simulink model "Tricopter_Controlled"  (R2015a)
settings: Solver=ode3  SolverMode=SingleTasking  StartTime=0.0  StopTime=inf  FixedStep=T_sim  RelTol=1e-3
values from neighbouring files (symbols this model uses):
  A_l_max_x = sqrt( (A_z_max)^2  -  g^2  )    [Run3Copter.m]
  A_l_max_y = g*tand(15)    [Run3Copter.m]
  A_z_max = Max_Thrust*3/m    [Run3Copter.m]
  Alt_0 = input(' Give the initial altitude (m): ')    [Run3Copter.m]
  B_hover_4dof = [-0.192641491537 -0.295051706147 -72.3190840892 -0.00308714144823 24.9504828653 -1.18743631629 9.87469464114e-05 6.48783896558 -0.0529805907426 -0.000387203135788 0.131620058452 2.24065603044 ... (54 elements, 6x9)]    [Effectiv_matrices.mat]
  CG_0 = [0,0,0.02]'    [SetupComplete.m]
  epsilon = 0.01    [Run3Copter.m]
  eta_23 = deg2rad(-1.3)    [Run3Copter.m]
  g = 9.81    [SetupComplete.m]
  h = 0.08    [SetupComplete.m]
  h_M = 0.064    [SetupComplete.m]
  Hover_eta_23 = deg2rad(-1.3)    [Run3Copter.m]
  Hover_throtle_1 = 0.745    [Run3Copter.m]
  Hover_throtle_23 = Hover_throtle_1/cos(Hover_eta_23)    [Run3Copter.m]
  I_BAC_0 = [ Ix,0,Ixz;0,Iy,0;Ixz,0,Iz]    [SetupComplete.m]
  Initial_Omegas = Omega_hover    [Run3Copter.m]
  Initial_Torques = Torque_hover    [Run3Copter.m]
  Ix = 0.103    [SetupComplete.m]
  Iy = 0.147    [SetupComplete.m]
  Iz = 0.237    [SetupComplete.m]
  l = 0.345    [SetupComplete.m]
  l_arm = 0.264    [SetupComplete.m]
  latitude = 52.071118    [Run3Copter.m]
  longitude = -0.627404    [Run3Copter.m]
  m = 3.51    [SetupComplete.m]
  m_0 = 2.61    [SetupComplete.m]
  m_M = 0.300    (= 0.3)    [SetupComplete.m]
  Rotation_sign = [ 1,-1,-1]    [SetupComplete.m]
  T_ctrl = 0.02    [Run3Copter.m]
  T_sim = 0.01    [Run3Copter.m]
  throtle_1 = 0*0.745    (= 0)    [Run3Copter.m]
  throtle_23 = throtle_1/cos(eta_23)    [Run3Copter.m]
  v_i0 = sqrt( 1/3*m*g/(2*rho*pi*R^2)  )    [SetupComplete.m]
undefined symbols (not defined in the file or in its folder): DOWN_0, EAST_0, Newton, NORTH_0, P_0, Q_0, R_0, Raphson, U_0, V_0, W_0
libraries: XXCopter_Control x64, simulink_extras x17, simulink x11, XXCopter x8
(part 3 of 6)

== system Tricopter_Controlled/TriCopter FCS/TriCopter FCS/Simulink_to_Px4 interface ==
  note: Terminal Debug Output
  note: RGB LED (uint8)
  note: Standard LED (Bool)
  note: PWM Output (uS)
  note: Enable Output (Bool)
  motors_signals : Inport
  servos_signals : Inport  Port=2
  pwm_arm : Inport  Port=3
  extern_signal_flihgt_mode : Inport  Port=4
  flight_mode : Inport  Port=5
  Bus Selector : BusSelector  OutputSignals=blue_LED,Red_LED,RGBLED.red,RGBLED.green,RGBLED.blue
  Data Type Conversion : DataTypeConversion  OutDataTypeStr=boolean
  Data Type Conversion1 : DataTypeConversion  OutDataTypeStr=boolean
  Data Type Conversion2 : DataTypeConversion  OutDataTypeStr=uint8
  Data Type Conversion3 : DataTypeConversion  OutDataTypeStr=uint8
  Data Type Conversion4 : DataTypeConversion  OutDataTypeStr=uint8
  Selector10 : Selector  InputPortWidth=6  Indices=4
  Selector11 : Selector  InputPortWidth=6  Indices=6
  Selector2 : Selector  InputPortWidth=3
  Selector3 : Selector  InputPortWidth=3  Indices=2
  Selector4 : Selector  InputPortWidth=3  Indices=3
  Selector5 : Selector  InputPortWidth=6  Indices=[1]
  Selector6 : Selector  InputPortWidth=6  Indices=[3]
  Selector8 : Selector  InputPortWidth=6  Indices=5
  Selector9 : Selector  InputPortWidth=6  Indices=[2]
  pwm1 : Outport  PortDimensions=1  SampleTime=T_ctrl
  pwm2 : Outport  Port=2  PortDimensions=1  SampleTime=T_ctrl
  pwm3 : Outport  Port=3  PortDimensions=1  SampleTime=T_ctrl
  pwm4 : Outport  Port=4  PortDimensions=1  SampleTime=T_ctrl
  pwm5 : Outport  Port=5  PortDimensions=1  SampleTime=T_ctrl
  pwm6 : Outport  Port=6  PortDimensions=1  SampleTime=T_ctrl
  pwm7 : Outport  Port=7  PortDimensions=1  SampleTime=T_ctrl
  pwm8 : Outport  Port=8  PortDimensions=1  SampleTime=T_ctrl
  pwm_arm1 : Outport  Port=9  PortDimensions=1  SampleTime=T_ctrl
  led_blue : Outport  Port=10  OutDataTypeStr=boolean  PortDimensions=1  SampleTime=T_ctrl
  led_red : Outport  Port=11  OutDataTypeStr=boolean  PortDimensions=1  SampleTime=T_ctrl
  rgb_red : Outport  Port=12  OutDataTypeStr=uint8  PortDimensions=1  SampleTime=T_ctrl
  rgb_green : Outport  Port=13  OutDataTypeStr=uint8  PortDimensions=1  SampleTime=T_ctrl
  rgb_blue : Outport  Port=14  OutDataTypeStr=uint8  PortDimensions=1  SampleTime=T_ctrl
  debug1 : Outport  Port=15  PortDimensions=1  SampleTime=T_ctrl
  debug2 : Outport  Port=16  PortDimensions=1  SampleTime=T_ctrl
  debug3 : Outport  Port=17  PortDimensions=1  SampleTime=T_ctrl
  debug4 : Outport  Port=18  PortDimensions=1  SampleTime=T_ctrl
  debug5 : Outport  Port=19  PortDimensions=1  SampleTime=T_ctrl
  debug6 : Outport  Port=20  PortDimensions=1  SampleTime=T_ctrl
  debug7 : Outport  Port=21  PortDimensions=1  SampleTime=T_ctrl
  debug8 : Outport  Port=22  PortDimensions=1  SampleTime=T_ctrl
  wires:
  motors_signals/1 -> Selector3/1, Selector4/1, Selector2/1
  servos_signals/1 -> Selector9/1, Selector5/1, Selector6/1, Selector10/1, Selector8/1, Selector11/1
  extern_signal_flihgt_mode/1 -> Bus Selector/1
  Bus Selector/2 -> Data Type Conversion1/1  "<Red_LED>"
  Selector2/1 -> pwm1/1
  Selector5/1 -> pwm2/1
  Selector9/1 -> pwm3/1
  Selector3/1 -> pwm4/1
  Selector6/1 -> pwm5/1
  Selector10/1 -> pwm6/1
  Selector4/1 -> pwm7/1
  Selector8/1 -> pwm8/1
  pwm_arm/1 -> pwm_arm1/1
  Bus Selector/3 -> Data Type Conversion2/1  "<red>"
  Bus Selector/4 -> Data Type Conversion3/1  "<green>"
  Bus Selector/5 -> Data Type Conversion4/1  "<blue>"
  flight_mode/1 -> debug8/1, debug7/1, debug6/1, debug5/1, debug4/1, debug3/1, debug1/1
  Data Type Conversion/1 -> led_blue/1
  Data Type Conversion1/1 -> led_red/1
  Data Type Conversion2/1 -> rgb_red/1
  Data Type Conversion3/1 -> rgb_green/1
  Data Type Conversion4/1 -> rgb_blue/1
  Selector11/1 -> debug2/1
  Bus Selector/1 -> Data Type Conversion/1  "<blue_LED>"

== system Tricopter_Controlled/TriCopter FCS/TriCopter FCS/Status signals ==
  flight_mode : Inport
  Not_allowed_change : Inport  Port=2
  Ground{,1..3} (4 alike) : Ground
  Beep : Outport
  Red_LED : Outport  Port=2
  blue_LED : Outport  Port=3
  blue_RGBLED : Outport  Port=4
  Red_RGBLED : Outport  Port=5
  green_RGBLED : Outport  Port=6
  wires:
  Ground/1 -> blue_RGBLED/1, Red_RGBLED/1, green_RGBLED/1
  Ground1/1 -> Beep/1
  Ground2/1 -> Red_LED/1
  Ground3/1 -> blue_LED/1

== system Tricopter_Controlled/TriCopter FCS/TriCopter FCS/flight_mode_effector ==
  flight_mode : Inport
  All_meas : Inport  Port=2
  Bus Creator : BusCreator  Inputs=6
  Bus Creator1 : BusCreator  Inputs=6
  Bus Selector1 : BusSelector  OutputSignals=Meas.Pos_meas_m,Params.V_yaw,Meas.Eulr_meas_rad,Meas.omega_b_meas_radps
  alt_act : Memory  X0=false  InheritSampleTime=on
  att_act : Memory  X0=false  InheritSampleTime=on
  flight_mode_effector : MATLAB Function  TreatAsAtomicUnit=on
  man_act : Memory  X0=false  InheritSampleTime=on
  pos_xy_act : Memory  X0=false  InheritSampleTime=on
  vel_yaw_xy_act : Memory  X0=false  InheritSampleTime=on
  vel_yaw_z_act : Memory  X0=false  InheritSampleTime=on
  Act_bus : Outport
  Controller_inits : Outport  Port=2  PortDimensions=12
  CA_reconf : Outport  Port=3
  Armed : Outport  Port=4
  wires:
  flight_mode/1 -> flight_mode_effector/1(flight_mode)
  flight_mode_effector/1(pos_xy_act) -> pos_xy_act/1
  flight_mode_effector/2(alt_act) -> alt_act/1
  flight_mode_effector/3(vel_yaw_xy_act) -> vel_yaw_xy_act/1
  flight_mode_effector/4(vel_yaw_z_act) -> vel_yaw_z_act/1
  flight_mode_effector/5(att_act) -> att_act/1
  flight_mode_effector/6(omega_b_act) -> man_act/1
  flight_mode_effector/9(vel_yaw_xy_init) -> Bus Creator1/3
  flight_mode_effector/12(b_rates_init) -> Bus Creator1/6
  flight_mode_effector/10(vel_yaw_z_init) -> Bus Creator1/4
  flight_mode_effector/11(att_init) -> Bus Creator1/5
  flight_mode_effector/7(pos_xy_init) -> Bus Creator1/1
  flight_mode_effector/8(alt_init) -> Bus Creator1/2
  Bus Selector1/2 -> flight_mode_effector/3(V_yaw)  "<V_yaw>"
  Bus Selector1/1 -> flight_mode_effector/2(X_e)  "<Pos_meas_m>"
  Bus Selector1/3 -> flight_mode_effector/4(Euler)  "<Eulr_meas_rad>"
  Bus Selector1/4 -> flight_mode_effector/5(omega_b)  "<omega_b_meas_radps>"
  pos_xy_act/1 -> Bus Creator/1  "pos_xy_act"
  alt_act/1 -> Bus Creator/2  "alt_act"
  vel_yaw_xy_act/1 -> Bus Creator/3  "vel_yaw_xy_act"
  vel_yaw_z_act/1 -> Bus Creator/4  "vel_yaw_z_act"
  att_act/1 -> Bus Creator/5  "att_act"
  man_act/1 -> Bus Creator/6  "omega_b_act"
  Bus Creator/1 -> Act_bus/1
  Bus Creator1/1 -> Controller_inits/1
  flight_mode_effector/13(CA_reconf) -> CA_reconf/1
  flight_mode_effector/14(Armed) -> Armed/1
  All_meas/1 -> Bus Selector1/1

== system Tricopter_Controlled/FlightGear visualization/Flat Earth to LLA/ne to lat//long/Latitude Between +//- 90  ==
  mu l : Inport
  Constant1 : Constant  Value=180
  Constant3 : Constant  Value=90
  Constant4 : Constant  Value=180
  Constant5 : Constant  Value=360
  Data Type Conversion : DataTypeConversion
  Demux : Demux  Outputs=2
  Gain : Gain  Gain=180
  Gain1 : Gain  Gain=2
  Gain2 : Gain  Gain=2
  Gain3 : Gain  Gain=360
  Gain4 : Gain  Gain=180
  Logical Operator1 : Logic  AllPortsSameDT=off  OutDataTypeStr=boolean
  Math Function1 : Math  Operator=rem  SaturateOnIntegerOverflow=on
  Math Function2 : Math  Operator=rem  SaturateOnIntegerOverflow=on
  Mux : Mux  Inputs=2
  Product : Product  Inputs=*/  RndMeth=Zero
  Product1 : Product  RndMeth=Zero
  Product2 : Product  Inputs=*/  RndMeth=Zero
  Product3 : Product  RndMeth=Zero
  Rounding Function : Rounding  Operator=fix
  Rounding Function1 : Rounding  Operator=fix
  Rounding Function2 : Rounding  Operator=fix
  Sum1 : Sum  Inputs=|-+
  Sum2 : Sum  Inputs=+--
  Sum3 : Sum  Inputs=++|
  sqrt : Sqrt  AlgorithmType=Newton-Raphson  SaturateOnIntegerOverflow=on
  "mu l " : Outport
  wires:
  Sum3/1 -> Mux/2
  Demux/2 -> Sum3/2
  Demux/1 -> Math Function1/1
  mu l/1 -> Demux/1
  Mux/1 -> "mu l "/1
  Constant1/1 -> Product/2
  Product/1 -> Rounding Function/1, Gain1/1
  Rounding Function/1 -> Gain/1
  Gain/1 -> Sum2/2
  Sum2/1 -> Mux/1
  Constant3/1 -> Math Function2/2
  Math Function2/1 -> Product3/2
  Product3/1 -> Sum2/3
  Rounding Function2/1 -> Gain2/1
  Gain2/1 -> Product3/1, Logical Operator1/1, Logical Operator1/2
  Product1/1 -> sqrt/1
  sqrt/1 -> Rounding Function2/1
  Constant4/1 -> Product2/2
  Product2/1 -> Rounding Function1/1
  Rounding Function1/1 -> Gain3/1
  Gain3/1 -> Sum1/1
  Math Function1/1 -> Sum1/2, Product2/1
  Sum1/1 -> Math Function2/1, Product/1, Sum2/1
  Constant5/1 -> Math Function1/2
  Logical Operator1/1 -> Data Type Conversion/1
  Gain4/1 -> Sum3/1
  Data Type Conversion/1 -> Gain4/1
  Gain1/1 -> Product1/2, Product1/1

== system Tricopter_Controlled/FlightGear visualization/Flat Earth to LLA/ne to lat//long/LongLat_offset  ==
  XY : Inport
  mu : Inport  Port=2
  " " : Trigonometry
  "  " : Trigonometry  Operator=cos
  Demux : Demux  Outputs=2
  "Find Radian/Distance " : Subsystem  TreatAsAtomicUnit=on
  Mux : Mux  Inputs=2
  Sum : Sum  Inputs=|+-
  Sum1 : Sum  Inputs=|++
  deg2rad : Gain  Gain=pi/180  SaturateOnIntegerOverflow=on  OutDataTypeStr=Inherit: Same as input  ParamDataTypeStr=Inherit: Same as input
  rad lat : Product  RndMeth=Zero
  "rad long " : Product  RndMeth=Zero
  ref_pos : Constant  Value=0
  x*cos : Product  RndMeth=Zero
  x*sin : Product  RndMeth=Zero
  y*cos : Product  RndMeth=Zero
  y*sin : Product  RndMeth=Zero
  DeltaLL_rad : Outport
  wires:
  mu/1 -> "Find Radian/Distance "/1(mu)
  "Find Radian/Distance "/1(dNorth) -> rad lat/2
  "Find Radian/Distance "/2(dEast) -> "rad long "/1
  rad lat/1 -> Mux/1
  "rad long "/1 -> Mux/2
  Mux/1 -> DeltaLL_rad/1
  deg2rad/1 -> "  "/1, " "/1
  Demux/2 -> y*cos/1, y*sin/1
  Sum1/1 -> "rad long "/2
  y*cos/1 -> Sum1/2
  x*sin/1 -> Sum1/1
  Sum/1 -> rad lat/1
  y*sin/1 -> Sum/2
  " "/1 -> x*sin/2, y*sin/2
  x*cos/1 -> Sum/1
  "  "/1 -> y*cos/2, x*cos/2
  Demux/1 -> x*sin/1, x*cos/1
  XY/1 -> Demux/1
  ref_pos/1 -> deg2rad/1

== system Tricopter_Controlled/FlightGear visualization/Flat Earth to LLA/ne to lat//long/Longitude Between +//-180  ==
  mu l : Inport
  Constant : Constant  Value=180
  Constant2 : Constant  Value=360
  Demux1 : Demux  Outputs=2
  Gain : Gain  Gain=360
  Math Function2 : Math  Operator=rem  SaturateOnIntegerOverflow=on
  Mux1 : Mux  Inputs=2
  Product : Product  Inputs=*/  RndMeth=Zero
  Rounding Function : Rounding  Operator=fix
  Sum2 : Sum  Inputs=|-+
  "mu l " : Outport
  wires:
  Mux1/1 -> "mu l "/1
  Demux1/1 -> Mux1/1
  mu l/1 -> Demux1/1
  Constant/1 -> Product/2
  Product/1 -> Rounding Function/1
  Rounding Function/1 -> Gain/1
  Gain/1 -> Sum2/1
  Sum2/1 -> Mux1/2
  Demux1/2 -> Math Function2/1
  Constant2/1 -> Math Function2/2
  Math Function2/1 -> Product/1, Sum2/2

== system Tricopter_Controlled/TriCopter FCS/Simulink to px4 input/Flat Earth to LLA/ne to lat//long ==
  Xe : Inport
  Demux : Demux  Outputs=2
  "Latitude Between +/- 90 " : Subsystem  TreatAsAtomicUnit=on
  "LongLat_offset " : Subsystem  TreatAsAtomicUnit=on
  "Longitude Between +/-180 " : Subsystem  TreatAsAtomicUnit=on
  Sel1 : Selector  InputPortWidth=3  Indices=[1,2]
  Sum2 : Sum  Inputs=++|
  initial_latg : Constant  Value=latitude
  initial_pos : Constant  Value=[latitude,longitude]
  rad2deg : Gain  Gain=180/pi  SaturateOnIntegerOverflow=on  OutDataTypeStr=Inherit: Same as input  ParamDataTypeStr=Inherit: Same as input
  lat_deg : Outport
  long_deg : Outport  Port=2
  wires:
  Xe/1 -> Sel1/1
  Sum2/1 -> "Latitude Between +/- 90 "/1(mu l)
  "LongLat_offset "/1(DeltaLL_rad) -> rad2deg/1
  Sel1/1 -> "LongLat_offset "/1(XY)
  rad2deg/1 -> Sum2/2
  initial_pos/1 -> Sum2/1
  initial_latg/1 -> "LongLat_offset "/2(mu)
  "Latitude Between +/- 90 "/1("mu l ") -> "Longitude Between +/-180 "/1(mu l)
  "Longitude Between +/-180 "/1("mu l ") -> Demux/1
  Demux/1 -> lat_deg/1
  Demux/2 -> long_deg/1

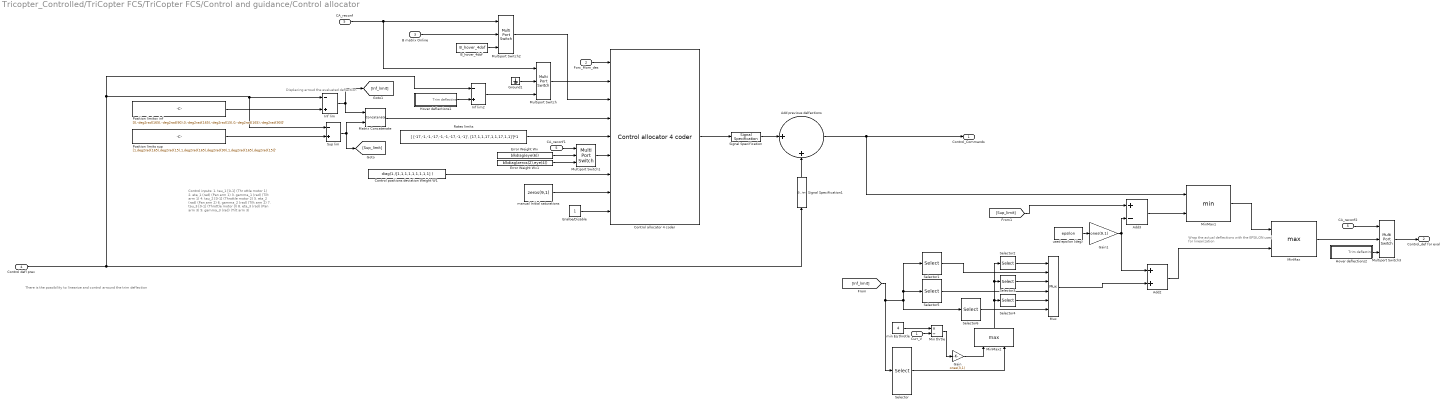
== system Tricopter_Controlled/TriCopter FCS/TriCopter FCS/Control and guidance/Control allocator ==
  note: There is the possibility to linearize and control arround the trim deflection
  note: Wrap the actual deflections with the EPSILON
      |  used for linearization
  note: Displacing arroud the evaluated deflection
  note: Control inputs:
      | 1. tau_1 [0-1] (Thr ottle motor 1)
      | 2. eta_1 (rad)  (Pan arm 1)
      | 3. gamma_1 (rad)  (Tilt arm 1)
      |
      | 4. tau_2 [0-1] (Throttle motor 2)
      | 5. eta_2 (rad)  (Pan arm 2)
      | 6. gamma_2 (rad)  (Tilt arm 2)
      |
      | 7. tau_3 [0-1] (Throttle motor 3)
      | 8. eta_3 (rad)  (Pan arm  3)
      | 9. gamma_3 (rad)  (Tilt arm 3)
  Curr_V : Inport
  Forc_Mom_des : Inport  Port=2
  B matrix Online : Inport  Port=3
  Control defl prev : Inport  Port=4
  CA_reconf : Inport  Port=5
  Add previous delfections : Sum  Inputs=|++
  Add2 : Sum
  Add3 : Sum  Inputs=+-
  B_hover_4dof : Constant  Value=B_hover_4dof
  CA_reconf1 : InportShadow  Port=5
  CA_reconf2 : InportShadow  Port=5
  Control allocator 4 coder : XXCopter_Control/Control allocator 4 coder  gamma=1  imax=50  T=T_ctrl
  Control positions deviation Weight W1 : Constant  Value=diag(1./[1,1,1,1,1,1,1,1,1] )
  Enalbe/Disable : Constant
  Error Weight Wv : Constant  Value=blkdiag(eye(6))
  Error Weight Wv1 : Constant  Value=blkdiag(zeros(2),eye(4))
  Gain : Gain  Gain=ones(3,1)
  Gain1 : Gain  Gain=ones(9,1)
  Ground1 : Ground
  Hover deflections1 : Subsystem  TreatAsAtomicUnit=on
  Hover deflections2 : Subsystem  TreatAsAtomicUnit=on
  Inf lim : Sum  Inputs=-+
  Inf lim2 : Sum  Inputs=-+
  Matrix Concatenate : Concatenate  Mode=Multidimensional array  ConcatenateDimension=2
  Min thrtle : Product  Inputs=*/
  MinMax : MinMax  Function=max  Inputs=2
  MinMax1 : MinMax  Inputs=2
  MinMax2 : MinMax  Function=max  Inputs=2
  Multiport Switch{,1..3} (4 alike) : MultiPortSwitch  Inputs=2
  Mux : Mux  Inputs=[1,2,1,2,1,2]
  Position limits sup : Constant  Value=[1,deg2rad(165),deg2rad(15),1,deg2rad(165),deg2rad(90),1,deg2rad(165),deg2rad(15)]'
  Position limitsv inf : Constant  Value=[0,-deg2rad(165),-deg2rad(90),0,-deg2rad(165),-deg2rad(15),0,-deg2rad(165),-deg2rad(90)]'
  Rates limits : Constant  Value=[ [-17,-1,-1,-17,-1,-1,-17,-1,-1]', [17,1,1,17,1,1,17,1,1]']*1
  Selector : Selector  InputPortWidth=9  Indices=[1,4,7]
  Selector1 : Selector  InputPortWidth=9  Indices=[2,3]
  Selector2 : Selector  InputPortWidth=3
  Selector3 : Selector  InputPortWidth=3
  Selector4 : Selector  InputPortWidth=3
  Selector5 : Selector  InputPortWidth=9  Indices=[2,3]
  Selector6 : Selector  InputPortWidth=9  Indices=[2,3]
  Signal Specification : SignalSpecification  Dimensions=[9,1]
  Signal Specification1 : SignalSpecification  Dimensions=[9,1]
  Sup lim : Sum  Inputs=-+
  manual Initial saturations : Constant  Value=zeros(9,1)
  min Eq throtle : Constant  Value=4
  used epsilon (deg) : Constant  Value=epsilon
  Control_Commands : Outport
  Control_def for eval : Outport  Port=2
  wires:
  MinMax1/1 -> MinMax/1
  Add3/1 -> MinMax1/2
  used epsilon (deg)/1 -> Gain1/1
  Gain1/1 -> Add2/1, Add3/2
  Add2/1 -> MinMax/2
  Control positions deviation Weight W1/1 -> Control allocator 4 coder/7
  Control allocator 4 coder/1 -> Signal Specification/1
  Enalbe/Disable/1 -> Control allocator 4 coder/9
  manual Initial saturations/1 -> Control allocator 4 coder/8
  Sup lim/1 -> [Sup_limit], Matrix Concatenate/2
  Inf lim/1 -> [Inf_limit], Matrix Concatenate/1
  Position limitsv inf/1 -> Inf lim/2
  Position limits sup/1 -> Sup lim/2
  Rates limits/1 -> Control allocator 4 coder/5
  Add previous delfections/1 -> Control_Commands/1, MinMax1/1
  Multiport Switch2/1 -> Control allocator 4 coder/3
  Signal Specification/1 -> Add previous delfections/1
  Signal Specification1/1 -> Add previous delfections/2
  Forc_Mom_des/1 -> Control allocator 4 coder/1
  Matrix Concatenate/1 -> Control allocator 4 coder/4
  Multiport Switch/1 -> Control allocator 4 coder/2
  Control defl prev/1 -> Signal Specification1/1, Inf lim/1, Sup lim/1, Inf lim2/1
  CA_reconf/1 -> Multiport Switch2/1, Multiport Switch/1
  B matrix Online/1 -> Multiport Switch2/2
  Ground1/1 -> Multiport Switch/2
  Inf lim2/1 -> Multiport Switch/3
  Hover deflections1/1(Trim deflectins) -> Inf lim2/2
  Multiport Switch3/1 -> Control_def for eval/1
  CA_reconf2/1 -> Multiport Switch3/1
  Hover deflections2/1(Trim deflectins) -> Multiport Switch3/3
  MinMax/1 -> Multiport Switch3/2
  B_hover_4dof/1 -> Multiport Switch2/3
  Multiport Switch1/1 -> Control allocator 4 coder/6
  CA_reconf1/1 -> Multiport Switch1/1
  Error Weight Wv/1 -> Multiport Switch1/2
  Error Weight Wv1/1 -> Multiport Switch1/3
  [Inf_limit] -> Selector5/1, Selector1/1, Selector6/1, Selector/1
  Selector/1 -> MinMax2/2
  min Eq throtle/1 -> Min thrtle/1
  Curr_V/1 -> Min thrtle/2
  Min thrtle/1 -> Gain/1
  Gain/1 -> MinMax2/1
  Selector2/1 -> Mux/1
  MinMax2/1 -> Selector4/1, Selector3/1, Selector2/1
  Selector3/1 -> Mux/3
  Selector4/1 -> Mux/5
  Selector1/1 -> Mux/2
  Selector5/1 -> Mux/4
  Selector6/1 -> Mux/6
  Mux/1 -> Add2/2
  [Sup_limit] -> Add3/1

== system Tricopter_Controlled/TriCopter FCS/TriCopter FCS/Control and guidance/Inner PI Controller Quaternions ==
  Accels ref (m/s^2) : Inport
  Phi_ref (rad) : Inport  Port=2
  Theta_ref (rad) : Inport  Port=3
  Yaw_ref (rad) : Inport  Port=4
  omega_b_ref_radps : Inport  Port=5
  All meas : Inport  Port=6
  activation_bus : Inport  Port=7
  init_cond : Inport  Port=8
  Add : Sum
  Add1 : Sum  Inputs=+-
  Add2 : Sum  Inputs=+-
  All meas1 : InportShadow  Port=6
  Attitude Controller : Subsystem
  Body Rates Controller : Subsystem
  Bus Selector : BusSelector  OutputSignals=Meas.Eulr_meas_rad
  Bus Selector1 : BusSelector  OutputSignals=Meas.q_meas
  Bus Selector2 : BusSelector  OutputSignals=att_act,omega_b_act
  Demux : Demux  Outputs=3
  Get Quaternion from des euler : MATLAB Function  TreatAsAtomicUnit=on
  Limits in Ang accel : Subsystem  TreatAsAtomicUnit=on
  Logical Operator2 : Logic  Operator=NOT  IconShape=distinctive  AllPortsSameDT=off  OutDataTypeStr=boolean
  Logical Operator3 : Logic  IconShape=distinctive  AllPortsSameDT=off  OutDataTypeStr=boolean
  MATLAB Function : MATLAB Function  TreatAsAtomicUnit=on
  Memory : Memory
  Mux : Mux  Inputs=2
  Quaternion_dot : MATLAB Function  TreatAsAtomicUnit=on  VariantControl=Variant
  Saturation1 : Saturate  UpperLimit=deg2rad(50)*[1,10,0.5]'  LowerLimit=-deg2rad(50)*[1,10,0.5]'
  Switch1 : Switch  Criteria=u2 ~= 0
  T : Gain  Gain=T_ctrl
  Accs_Ang_acc des : Outport
  wires:
  Accels ref (m/s^2)/1 -> Mux/1
  Mux/1 -> Accs_Ang_acc des/1
  All meas/1 -> Bus Selector/1, Attitude Controller/5(All_meas)
  Bus Selector/1 -> Limits in Ang accel/2(Euler meas), MATLAB Function/2(Euler)  "<Eulr_meas_rad>"
  Demux/1 -> Body Rates Controller/1(p_ref)
  Demux/2 -> Body Rates Controller/2(q_ref)
  Demux/3 -> Body Rates Controller/3(r_ref)
  Phi_ref (rad)/1 -> Attitude Controller/2(Phi_ref (rad)), Get Quaternion from des euler/1(phi)
  Theta_ref (rad)/1 -> Get Quaternion from des euler/2(theta)
  Yaw_ref (rad)/1 -> Attitude Controller/4(Yaw_ref (rad)), Get Quaternion from des euler/3(psi)
  Bus Selector1/1 -> Quaternion_dot/2(q)  "<q_meas>"
  Get Quaternion from des euler/1(q) -> Attitude Controller/3(q_ref)
  Attitude Controller/1(quat_dot des (rad/s)) -> Quaternion_dot/1(q_dot)
  Limits in Ang accel/1(ang Ace des) -> Add2/1, Mux/2
  Switch1/1 -> Add1/2, Saturation1/1
  Body Rates Controller/1(Angular acc des (rad/s^2)) -> Add2/2, Limits in Ang accel/1(Ang Ace des)
  Add/1 -> MATLAB Function/1(omega_b)
  Add2/1 -> T/1
  Add1/1 -> Add/2
  T/1 -> Add/1
  MATLAB Function/1(Euler_dot) -> Memory/1
  init_cond/1 -> Body Rates Controller/5(init_cond), Attitude Controller/7(init_cond)
  activation_bus/1 -> Attitude Controller/6(activation_bus), Bus Selector2/1, Body Rates Controller/6(activation_bus)
  All meas1/1 -> Body Rates Controller/4(All_meas), Bus Selector1/1
  Bus Selector2/1 -> Logical Operator2/1  "<att_act>"
  Logical Operator2/1 -> Logical Operator3/1
  Bus Selector2/2 -> Logical Operator3/2  "<omega_b_act>"
  Saturation1/1 -> Demux/1, Add1/1
  Logical Operator3/1 -> Switch1/2
  Quaternion_dot/1(omega_b) -> Switch1/3
  omega_b_ref_radps/1 -> Switch1/1
  Memory/1 -> Attitude Controller/1(AWU)

== system Tricopter_Controlled/TriCopter FCS/TriCopter FCS/Control and guidance/NDI ==
  note: Rejection for the
      | angular accelerations
  note: Pseudo control inputs:
      | 1. Desired angular accelerations (rad/s^2)
      | 2. Desired accelerations (m/s^2) in body axes
  pseudo_control (m/s^2;rad/s^2) : Inport
  Control_defl for eval : Inport  Port=2
  All_meas : Inport  Port=3
  3Copter_4_NDI&CA : Subsystem  TreatAsAtomicUnit=on
  Bus Selector : BusSelector  OutputSignals=Meas.omega_b_meas_radps,Meas.q_meas,Meas.V_b_meas,Meas.Alt_meas_m,Meas.Volt
  Demux : Demux  Outputs=[3,3]
  Derivative1 : Derivative  CoefficientInTFapproximation=500
  Ground : Ground
  Ground1 : Ground
  Inversion : Sum  Inputs=|+-
  Mux : Mux  Inputs=[3,3]
  Mux2 : Mux  Inputs=[3,3]
  Rot eqs_ Get moments : XXCopter_Control/Rot eqs_ Get moments
  Transl Eqs_ Get forces : XXCopter_Control/Transl Eqs_ Get forces
  "angles " : Selector  IndexMode=Zero-based  InputPortWidth=9  Indices=[1,2,4,5,7,8]
  epsilon (rad or unitary) : Constant  Value=epsilon
  m : Constant  Value=m
  m1 : Constant  Value=m
  Virtual Control Commands : Outport
  B online : Outport  Port=2
  Control_defl eval (rad) : Outport  Port=3
  wires:
  3Copter_4_NDI&CA/3(CA_grad) -> B online/1
  Mux/1 -> Inversion/1
  Mux2/1 -> Inversion/2  "f_x(x)"
  All_meas/1 -> Bus Selector/1
  pseudo_control (m/s^2;rad/s^2)/1 -> Demux/1
  Demux/2 -> Rot eqs_ Get moments/2, Transl Eqs_ Get forces/4
  Demux/1 -> Transl Eqs_ Get forces/1
  Bus Selector/1 -> Transl Eqs_ Get forces/3, Rot eqs_ Get moments/1, 3Copter_4_NDI&CA/6(omega_b)  "<omega_b_meas_radps>"
  Bus Selector/3 -> Transl Eqs_ Get forces/2, 3Copter_4_NDI&CA/4(Vb)  "<V_b_meas>"
  3Copter_4_NDI&CA/4(I_BAC) -> Rot eqs_ Get moments/3
  3Copter_4_NDI&CA/5("CG ") -> Transl Eqs_ Get forces/6
  Control_defl for eval/1 -> 3Copter_4_NDI&CA/2(Control Inputs (rad)), Control_defl eval (rad)/1, "angles "/1
  Bus Selector/4 -> 3Copter_4_NDI&CA/3(h)  "<Alt_meas_m>"
  Bus Selector/2 -> 3Copter_4_NDI&CA/5(q)  "<q_meas>"
  m1/1 -> 3Copter_4_NDI&CA/11(" m")
  m/1 -> Transl Eqs_ Get forces/5
  epsilon (rad or unitary)/1 -> 3Copter_4_NDI&CA/1("epsilon (rad or unitary) ")
  Transl Eqs_ Get forces/1 -> Mux/1
  Rot eqs_ Get moments/1 -> Mux/2
  3Copter_4_NDI&CA/1(Forces) -> Mux2/1
  3Copter_4_NDI&CA/2(Moments) -> Mux2/2
  Inversion/1 -> Virtual Control Commands/1
  Ground/1 -> 3Copter_4_NDI&CA/7(Omegas_dot_actual)
  "angles "/1 -> Derivative1/1, 3Copter_4_NDI&CA/8(angles_actual)
  Derivative1/1 -> 3Copter_4_NDI&CA/9(angles_dot_actual)
  Ground1/1 -> 3Copter_4_NDI&CA/10(angles_dot_dot_actual)
  Bus Selector/5 -> 3Copter_4_NDI&CA/12(Curr_V)  "<Volt>"

== system Tricopter_Controlled/TriCopter FCS/TriCopter FCS/Control and guidance/Otter Overactuated P Controller ==
  Position ref (m) : Inport
  Vel_yaw_ref(m) : Inport  Port=2
  All meas : Inport  Port=3
  activation_bus : Inport  Port=4
  init_cond : Inport  Port=5
  AWU : Product  Multiplication=Matrix(*)
  Add : Sum
  Add1 : Sum  Inputs=+-
  Add2 : Sum  Inputs=+-
  Bus Selector1 : BusSelector  OutputSignals=Params.T_Fe_Fyaw,Params.V_yaw,Params.DCM
  Bus Selector2 : BusSelector  OutputSignals=pos_xy_act,vel_yaw_xy_act,alt_act,vel_yaw_z_act
  Demux1 : Demux  Outputs=3
  Demux2 : Demux  Outputs=3
  Demux3 : Demux  Outputs=[2,1]
  Logical Operator : Logic  IconShape=distinctive  AllPortsSameDT=off  OutDataTypeStr=boolean
  Logical Operator1 : Logic  Operator=NOT  IconShape=distinctive  AllPortsSameDT=off  OutDataTypeStr=boolean
  Logical Operator2 : Logic  Operator=NOT  IconShape=distinctive  AllPortsSameDT=off  OutDataTypeStr=boolean
  Logical Operator3 : Logic  IconShape=distinctive  AllPortsSameDT=off  OutDataTypeStr=boolean
  Matrix Multiply1 : Product  Multiplication=Matrix(*)
  Matrix Multiply2 : Product  Multiplication=Matrix(*)
  Matrix Multiply3 : Product  Multiplication=Matrix(*)
  Memory : Memory
  Mux : Mux  Inputs=[2,1]
  Permute Dimensions : PermuteDimensions
  Permute Dimensions1 : PermuteDimensions
  Permute Dimensions2 : PermuteDimensions
  Position Controller : Subsystem
  Saturation : Saturate  UpperLimit=[A_l_max_x,A_l_max_y,g]  LowerLimit=-[A_l_max_x,A_l_max_y,A_z_max-g]
  Saturation1 : Saturate  UpperLimit=[10,10,v_i0]'  LowerLimit=-[10,10,2*v_i0]'
  Selector : Selector  InputPortWidth=3  Indices=[1,2]
  Selector1 : Selector  InputPortWidth=3  Indices=3
  Switch : Switch  Criteria=u2 ~= 0
  Switch1 : Switch  Criteria=u2 ~= 0
  T : Gain  Gain=T_ctrl
  Velocity Controller : Subsystem
  activation_bus1 : InportShadow  Port=4
  init_cond1 : InportShadow  Port=5
  Accels des : Outport
  wires:
  Demux2/3 -> Velocity Controller/3(Vyaw_z_ref)
  Demux2/1 -> Velocity Controller/1(Vyaw_x_ref)
  Demux2/2 -> Velocity Controller/2(Vyaw_y_ref)
  All meas/1 -> Position Controller/6(All_meas), Bus Selector1/1
  Position ref (m)/1 -> Demux1/1
  Demux1/3 -> Position Controller/4(X_e_z_ref)
  Demux1/2 -> Position Controller/3(X_e_y_ref)
  Demux1/1 -> Position Controller/2(X_e_x_ref)
  Bus Selector1/3 -> Permute Dimensions/1  "<DCM>"
  Matrix Multiply1/1 -> Accels des/1
  Permute Dimensions/1 -> Matrix Multiply1/1
  Position Controller/1(Ve des (m/s)) -> Matrix Multiply2/2
  Saturation1/1 -> Add1/1, Demux2/1
  Saturation/1 -> Add2/1, Matrix Multiply3/2
  Bus Selector1/1 -> Permute Dimensions2/1, Matrix Multiply2/1, Permute Dimensions1/1  "<T_Fe_Fyaw>"
  Mux/1 -> Add1/2, Saturation1/1
  Matrix Multiply3/1 -> Matrix Multiply1/2  "in F_e"
  Permute Dimensions1/1 -> Matrix Multiply3/1
  Velocity Controller/1(Acc_yaw des (m/s)) -> Add2/2, Saturation/1
  Permute Dimensions2/1 -> AWU/1
  Add/1 -> AWU/2
  Add2/1 -> T/1
  Add1/1 -> Add/2
  AWU/1 -> Memory/1
  T/1 -> Add/1
  activation_bus/1 -> Bus Selector2/1, Position Controller/5(activation_bus)
  activation_bus1/1 -> Velocity Controller/5(activation_bus)
  init_cond/1 -> Position Controller/7(init_cond)
  Bus Selector1/2 -> Velocity Controller/4(V_yaw_meas)  "<V_yaw>"
  Matrix Multiply2/1 -> Demux3/1
  Switch/1 -> Mux/1
  Demux3/1 -> Switch/3
  Vel_yaw_ref(m)/1 -> Selector/1, Selector1/1
  Selector/1 -> Switch/1
  Switch1/1 -> Mux/2
  Demux3/2 -> Switch1/3
  Selector1/1 -> Switch1/1
  init_cond1/1 -> Velocity Controller/6(Init_cond)
  Bus Selector2/1 -> Logical Operator1/1  "<pos_xy_act>"
  Bus Selector2/3 -> Logical Operator2/1  "<alt_act>"
  Logical Operator1/1 -> Logical Operator/1
  Bus Selector2/2 -> Logical Operator/2  "<vel_yaw_xy_act>"
  Logical Operator2/1 -> Logical Operator3/1
  Bus Selector2/4 -> Logical Operator3/2  "<vel_yaw_z_act>"
  Logical Operator/1 -> Switch/2
  Logical Operator3/1 -> Switch1/2
  Memory/1 -> Position Controller/1(AWU)

== system Tricopter_Controlled/TriCopter FCS/TriCopter FCS/Control and guidance/keep -90//90 ==
  in (rad) : Inport
  Constant : Constant  Value=180
  Constant2 : Constant  Value=360
  Gain : Gain  Gain=360
  Math Function2 : Math  Operator=rem  SaturateOnIntegerOverflow=on
  Product : Product  Inputs=*/  RndMeth=Zero
  Rounding Function : Rounding  Operator=fix
  Sum2 : Sum  Inputs=|-+
  deg2rad1 : Gain  Gain=pi/180  SaturateOnIntegerOverflow=on  OutDataTypeStr=Inherit: Same as input  ParamDataTypeStr=Inherit: Same as input
  rad2deg : Gain  Gain=180/pi  SaturateOnIntegerOverflow=on  OutDataTypeStr=Inherit: Same as input  ParamDataTypeStr=Inherit: Same as input
  out (rad) : Outport
  wires:
  deg2rad1/1 -> out (rad)/1
  Sum2/1 -> deg2rad1/1
  Math Function2/1 -> Sum2/2, Product/1
  Constant2/1 -> Math Function2/2
  rad2deg/1 -> Math Function2/1
  Gain/1 -> Sum2/1
  Rounding Function/1 -> Gain/1
  Product/1 -> Rounding Function/1
  Constant/1 -> Product/2
  in (rad)/1 -> rad2deg/1

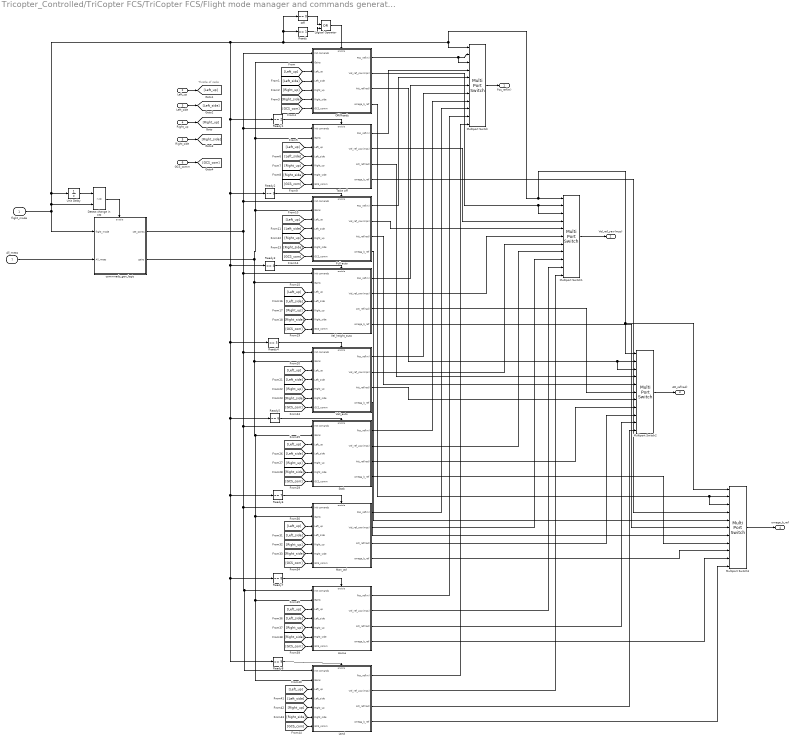
== system Tricopter_Controlled/TriCopter FCS/TriCopter FCS/Flight mode manager and commands generator/Commands generator ==
  note: Throtle of radio
  flight_mode : Inport
  Left_up : Inport  Port=2
  Left_side : Inport  Port=3
  Right_up : Inport  Port=4
  Right_side : Inport  Port=5
  GCS_comm : Inport  Port=6
  All_meas : Inport  Port=7
  Detect change in FM : RelationalOperator  Operator=~=  OutDataTypeStr=boolean
  Full auto : Subsystem  TreatAsAtomicUnit=on
  Home : Subsystem  TreatAsAtomicUnit=on
  "Land " : Subsystem  TreatAsAtomicUnit=on
  Logical Operator : Logic  Operator=OR  IconShape=distinctive  AllPortsSameDT=off  OutDataTypeStr=boolean
  Man_ctrl : Subsystem  TreatAsAtomicUnit=on
  Multiport Switch{,1..3} (4 alike) : MultiPortSwitch  DataPortOrder=Zero-based contiguous  Inputs=10
  Off : simulink/Logic and Bit Operations/Compare To Constant  relop===  const=0  OutDataTypeStr=boolean
  Off/Ready : Subsystem  TreatAsAtomicUnit=on
  Ready : simulink/Logic and Bit Operations/Compare To Constant  relop===  const=1  OutDataTypeStr=boolean
  Ready1 : simulink/Logic and Bit Operations/Compare To Constant  relop===  const=2  OutDataTypeStr=boolean
  Ready2 : simulink/Logic and Bit Operations/Compare To Constant  relop===  const=3  OutDataTypeStr=boolean
  Ready3 : simulink/Logic and Bit Operations/Compare To Constant  relop===  const=4  OutDataTypeStr=boolean
  Ready4 : simulink/Logic and Bit Operations/Compare To Constant  relop===  const=5  OutDataTypeStr=boolean
  Ready5 : simulink/Logic and Bit Operations/Compare To Constant  relop===  const=6  OutDataTypeStr=boolean
  Ready6 : simulink/Logic and Bit Operations/Compare To Constant  relop===  const=7  OutDataTypeStr=boolean
  Ready7 : simulink/Logic and Bit Operations/Compare To Constant  relop===  const=8  OutDataTypeStr=boolean
  Ready8 : simulink/Logic and Bit Operations/Compare To Constant  relop===  const=9  OutDataTypeStr=boolean
  Stab : Subsystem  TreatAsAtomicUnit=on
  Take off : Subsystem  TreatAsAtomicUnit=on
  Unit Delay : UnitDelay  SampleTime=-1
  Vel_height_auto : Subsystem  TreatAsAtomicUnit=on
  Vell_auto : Subsystem  TreatAsAtomicUnit=on
  commnads_gen_logic : Subsystem
  Pos_ref(m) : Outport
  Vel_ref_yaw(mps) : Outport  Port=2
  Att_ref(rad) : Outport  Port=3
  omega_b_ref : Outport  Port=4
  wires:
  flight_mode/1 -> Detect change in FM/2, Unit Delay/1, Ready8/1, Ready7/1, Ready6/1, Ready5/1, Ready4/1, Ready3/1, Ready2/1, Ready1/1, Ready/1, Off/1, Multiport Switch2/1, Multiport Switch3/1, Multiport Switch1/1, Multiport Switch/1, commnads_gen_logic/1(flight_mode)
  Multiport Switch/1 -> Pos_ref(m)/1
  Multiport Switch1/1 -> Vel_ref_yaw(mps)/1
  Multiport Switch2/1 -> Att_ref(rad)/1
  Multiport Switch3/1 -> omega_b_ref/1
  Right_up/1 -> [Right_up]
  Left_up/1 -> [Left_up]
  Right_side/1 -> [Right_side]
  Left_side/1 -> [Left_side]
  GCS_comm/1 -> [GCS_com]
  [Left_up] -> Off/Ready/3(Left_up)
  [Left_side] -> Off/Ready/4(Left_side)
  [Right_up] -> Off/Ready/5(Right_up)
  [Right_side] -> Off/Ready/6(Right_side)
  [GCS_com] -> Off/Ready/7(GCS_comm)
  [Left_up] -> Take off/3(Left_up)
  [Left_side] -> Take off/4(Left_side)
  [Right_up] -> Take off/5(Right_up)
  [Right_side] -> Take off/6(Right_side)
  [GCS_com] -> Take off/7(GCS_comm)
  [Left_up] -> Full auto/3(Left_up)
  [Left_side] -> Full auto/4(Left_side)
  [Right_up] -> Full auto/5(Right_up)
  [Right_side] -> Full auto/6(Right_side)
  [GCS_com] -> Full auto/7(GCS_comm)
  [Left_up] -> Vel_height_auto/3(Left_up)
  [Left_side] -> Vel_height_auto/4(Left_side)
  [Right_up] -> Vel_height_auto/5(Right_up)
  [Right_side] -> Vel_height_auto/6(Right_side)
  [GCS_com] -> Vel_height_auto/7(GCS_comm)
  [Left_up] -> Vell_auto/3(Left_up)
  [Left_side] -> Vell_auto/4(Left_side)
  [Right_up] -> Vell_auto/5(Right_up)
  [Right_side] -> Vell_auto/6(Right_side)
  [GCS_com] -> Vell_auto/7(GCS_comm)
  [Left_up] -> Stab/3(Left_up)
  [Left_side] -> Stab/4(Left_side)
  [Right_up] -> Stab/5(Right_up)
  [Right_side] -> Stab/6(Right_side)
  [GCS_com] -> Stab/7(GCS_comm)
  [Left_up] -> Man_ctrl/3(Left_up)
  [Left_side] -> Man_ctrl/4(Left_side)
  [Right_up] -> Man_ctrl/5(Right_up)
  [Right_side] -> Man_ctrl/6(Right_side)
  [GCS_com] -> Man_ctrl/7(GCS_comm)
  [Left_up] -> Home/3(Left_up)
  [Left_side] -> Home/4(Left_side)
  [Right_up] -> Home/5(Right_up)
  [Right_side] -> Home/6(Right_side)
  [GCS_com] -> Home/7(GCS_comm)
  [Left_up] -> "Land "/3(Left_up)
  [Left_side] -> "Land "/4(Left_side)
  [Right_up] -> "Land "/5(Right_up)
  [Right_side] -> "Land "/6(Right_side)
  [GCS_com] -> "Land "/7(GCS_comm)
  Off/1 -> Logical Operator/1
  Ready/1 -> Logical Operator/2
  Logical Operator/1 -> Off/Ready/Enable
  Ready1/1 -> Take off/Enable
  Ready2/1 -> Full auto/Enable
  Ready3/1 -> Vel_height_auto/Enable
  Ready4/1 -> Vell_auto/Enable
  Ready5/1 -> Stab/Enable
  Ready6/1 -> Man_ctrl/Enable
  Ready7/1 -> Home/Enable
  Ready8/1 -> "Land "/Enable
  Off/Ready/1(Pos_ref(m)) -> Multiport Switch/3, Multiport Switch/2
  Take off/1(Pos_ref(m)) -> Multiport Switch/4
  Full auto/1(Pos_ref(m)) -> Multiport Switch/5
  Vel_height_auto/1(Pos_ref(m)) -> Multiport Switch/6
  Vell_auto/1(Pos_ref(m)) -> Multiport Switch/7
  Stab/1(Pos_ref(m)) -> Multiport Switch/8
  Man_ctrl/1(Pos_ref(m)) -> Multiport Switch/9
  Home/1(Pos_ref(m)) -> Multiport Switch/10
  "Land "/1(Pos_ref(m)) -> Multiport Switch/11
  Off/Ready/2(Vel_ref_yaw(mps)) -> Multiport Switch1/3, Multiport Switch1/2
  Take off/2(Vel_ref_yaw(mps)) -> Multiport Switch1/4
  Full auto/2(Vel_ref_yaw(mps)) -> Multiport Switch1/5
  Vel_height_auto/2(Vel_ref_yaw(mps)) -> Multiport Switch1/6
  Vell_auto/2(Vel_ref_yaw(mps)) -> Multiport Switch1/7
  Stab/2(Vel_ref_yaw(mps)) -> Multiport Switch1/8
  Man_ctrl/2(Vel_ref_yaw(mps)) -> Multiport Switch1/9
  Home/2(Vel_ref_yaw(mps)) -> Multiport Switch1/10
  "Land "/2(Vel_ref_yaw(mps)) -> Multiport Switch1/11
  Off/Ready/3(Att_ref(rad)) -> Multiport Switch2/3, Multiport Switch2/2
  Take off/3(Att_ref(rad)) -> Multiport Switch2/4
  Full auto/3(Att_ref(rad)) -> Multiport Switch2/5
  Vel_height_auto/3(Att_ref(rad)) -> Multiport Switch2/6
  Vell_auto/3(Att_ref(rad)) -> Multiport Switch2/7
  Stab/3(Att_ref(rad)) -> Multiport Switch2/8
  Man_ctrl/3(Att_ref(rad)) -> Multiport Switch2/9
  Home/3(Att_ref(rad)) -> Multiport Switch2/10
  "Land "/3(Att_ref(rad)) -> Multiport Switch2/11
  Off/Ready/4(omega_b_ref) -> Multiport Switch3/3, Multiport Switch3/2
  Take off/4(omega_b_ref) -> Multiport Switch3/4
  Full auto/4(omega_b_ref) -> Multiport Switch3/5
  Vel_height_auto/4(omega_b_ref) -> Multiport Switch3/6
  Vell_auto/4(omega_b_ref) -> Multiport Switch3/7
  Stab/4(omega_b_ref) -> Multiport Switch3/8
  Man_ctrl/4(omega_b_ref) -> Multiport Switch3/9
  Home/4(omega_b_ref) -> Multiport Switch3/10
  "Land "/4(omega_b_ref) -> Multiport Switch3/11
  commnads_gen_logic/2(gains) -> Full auto/2(Gains), Take off/2(Gains), Off/Ready/2(Gains), Stab/2(Gains), "Land "/2(Gains), Home/2(Gains), Man_ctrl/2(Gains), Vell_auto/2(Gains), Vel_height_auto/2(Gains)
  commnads_gen_logic/1(set_points) -> Take off/1(Init comands), Off/Ready/1(Init comands), Full auto/1(Init comands), Stab/1(Init comands), "Land "/1(Init comands), Home/1(Init comands), Man_ctrl/1(Init comands), Vell_auto/1(Init comands), Vel_height_auto/1(Init comands)
  All_meas/1 -> commnads_gen_logic/2(All_meas)
  Unit Delay/1 -> Detect change in FM/1
  Detect change in FM/1 -> commnads_gen_logic/Enable

== system Tricopter_Controlled/TriCopter FCS/TriCopter FCS/Flight mode manager and commands generator/Flight manager ==
  note: This guy should be able to overwrite any flghlit_mode at any moment
  flight_mode_request : Inport
  All_meas : Inport  Port=2
  Safety_stab_switch : Inport  Port=3
  Bus Selector : BusSelector  OutputSignals=Params.gps_pdop,Params.gps_sat,Meas.Pos_meas_m,Params.V_yaw,Meas.Eulr_meas_rad,Meas.Volt
  Bus Selector1 : BusSelector  OutputSignals=Params.gps_pdop,Params.gps_vdop,Params.gps_sat,Meas.Pos_meas_m,Meas.Volt,Params.a_meas
  Memory : Memory
  Parameters_based_decision_making : MATLAB Function  TreatAsAtomicUnit=on
  Selector : Selector  InputPortWidth=3  Indices=3
  Unary Minus : UnaryMinus
  flight_mode_manager : MATLAB Function  TreatAsAtomicUnit=on
  flight_mode : Outport
  not_allowed_transition : Outport  Port=2
  wires:
  flight_mode_request/1 -> flight_mode_manager/1(flight_mode_reqest)
  All_meas/1 -> Bus Selector1/1, Bus Selector/1
  flight_mode_manager/1(flight_mode_out) -> Parameters_based_decision_making/1(flight_mode)
  Parameters_based_decision_making/1(flight_mode_out) -> flight_mode/1, Memory/1
  Memory/1 -> flight_mode_manager/9(flight_mode)
  Safety_stab_switch/1 -> flight_mode_manager/2(Safety_stab_switch)
  Bus Selector/1 -> flight_mode_manager/3(p_dop)  "<gps_pdop>"
  Bus Selector/5 -> flight_mode_manager/7(Euler)  "<Eulr_meas_rad>"
  Bus Selector/4 -> flight_mode_manager/6(Vyaw)  "<V_yaw>"
  Bus Selector/3 -> flight_mode_manager/5(Xe)  "<Pos_meas_m>"
  Bus Selector/2 -> flight_mode_manager/4(num_sats)  "<gps_sat>"
  Bus Selector1/1 -> Parameters_based_decision_making/2(pdop)  "<gps_pdop>"
  Bus Selector1/2 -> Parameters_based_decision_making/3(vdop)  "<gps_vdop>"
  Bus Selector1/3 -> Parameters_based_decision_making/4(num_sats)  "<gps_sat>"
  Bus Selector1/5 -> Parameters_based_decision_making/6(Volt)  "<Volt>"
  Bus Selector1/6 -> Parameters_based_decision_making/7(Accs)  "<a_meas>"
  Selector/1 -> Unary Minus/1
  Bus Selector1/4 -> Selector/1  "<Pos_meas_m>"
  Unary Minus/1 -> Parameters_based_decision_making/5(Alt)
  Bus Selector/6 -> flight_mode_manager/8(Volt)  "<Volt>"
  flight_mode_manager/2(NOT_allowed_sign) -> not_allowed_transition/1

== system Tricopter_Controlled/TriCopter FCS/TriCopter FCS/Px4_to_simulink input interface/DCM1 ==
  Euler : Inport  PortDimensions=3
  Fcn11 : Fcn  Expr=u(5)*u(4)
  Fcn12 : Fcn  Expr=u(5)*u(1)
  Fcn13 : Fcn  Expr=-u(2)
  Fcn21 : Fcn  Expr=u(3)*u(2)*u(4) - u(6)*u(1)
  Fcn22 : Fcn  Expr=u(3)*u(2)*u(1) + u(6)*u(4)
  Fcn23 : Fcn  Expr=u(3)*u(5)
  Fcn31 : Fcn  Expr=u(6)*u(2)*u(4) + u(3)*u(1)
  Fcn32 : Fcn  Expr=u(6)*u(2)*u(1) - u(3)*u(4)
  Fcn33 : Fcn  Expr=u(6)*u(5)
  Mux : Mux  Inputs=2
  Mux1 : Mux  Inputs=9
  Reshape : Reshape  OutputDimensionality=Customize  OutputDimensions=[3,3]
  sincos : Trigonometry  Operator=sincos
  DCM : Outport  PortDimensions=[3,3]
  wires:
  Fcn33/1 -> Mux1/9
  Fcn32/1 -> Mux1/8
  Fcn23/1 -> Mux1/6
  Fcn22/1 -> Mux1/5
  Fcn31/1 -> Mux1/7
  Fcn21/1 -> Mux1/4
  Fcn13/1 -> Mux1/3
  Fcn12/1 -> Mux1/2
  Fcn11/1 -> Mux1/1
  Mux/1 -> Fcn22/1, Fcn23/1, Fcn31/1, Fcn33/1, Fcn32/1, Fcn21/1, Fcn13/1, Fcn12/1, Fcn11/1
  sincos/2 -> Mux/2
  sincos/1 -> Mux/1
  Reshape/1 -> DCM/1
  Euler/1 -> sincos/1
  Mux1/1 -> Reshape/1

== system Tricopter_Controlled/FlightGear visualization/Flat Earth to LLA/ne to lat//long/LongLat_offset /Find Radian//Distance  ==
  note: R
  mu : Inport
  Constant{,2..3,5..6} (5 alike) : Constant
  Constant1 : Constant  Value=6378137
  Constant4 : Constant  Value=1/298.257223563
  Product1 : Product  Inputs=*/  RndMeth=Zero
  Product2 : Product  RndMeth=Zero
  Product3 : Product  Inputs=**/  RndMeth=Zero
  Product4 : Product  RndMeth=Zero
  Product5 : Product  RndMeth=Zero
  Product6 : Product  Inputs=4  RndMeth=Zero
  Sum : Sum  Inputs=-+
  Sum1 : Sum  Inputs=|+-
  Sum2 : Sum  Inputs=|+-
  Sum3 : Sum  Inputs=|+-
  Trigonometric Function : Trigonometry  Operator=cos
  Trigonometric Function1 : Trigonometry  Operator=atan2
  Trigonometric Function2 : Trigonometry  Operator=atan2
  Trigonometric Function3 : Trigonometry
  deg2rad : Gain  Gain=pi/180  SaturateOnIntegerOverflow=on  OutDataTypeStr=Inherit: Same as input  ParamDataTypeStr=Inherit: Same as input
  f : Constant
  sqrt : Sqrt  AlgorithmType=Newton-Raphson  SaturateOnIntegerOverflow=on
  sqrt1 : Sqrt  AlgorithmType=Newton-Raphson  SaturateOnIntegerOverflow=on
  dNorth : Outport
  dEast : Outport  Port=2
  wires:
  Trigonometric Function2/1 -> dEast/1
  Trigonometric Function1/1 -> dNorth/1
  Constant3/1 -> Trigonometric Function2/1
  Constant2/1 -> Trigonometric Function1/1
  Product4/1 -> Trigonometric Function2/2
  mu/1 -> deg2rad/1
  Trigonometric Function/1 -> Product4/2
  Product3/1 -> Trigonometric Function1/2  "Rm"
  Sum1/1 -> Product3/2
  Product1/1 -> Product4/1, Product3/1  "Rn"
  Constant/1 -> Sum1/1
  Product2/1 -> Sum1/2
  Constant1/1 -> Product1/1
  sqrt/1 -> Product1/2
  Sum3/1 -> Product3/3, sqrt/1
  f/1 -> Sum/2
  Constant4/1 -> Sum/1
  Sum/1 -> Product5/1, Product5/2
  Product5/1 -> Sum2/2
  Constant5/1 -> Sum2/1
  Sum2/1 -> sqrt1/1
  deg2rad/1 -> Trigonometric Function3/1, Trigonometric Function/1
  Trigonometric Function3/1 -> Product6/4, Product6/3
  sqrt1/1 -> Product6/1, Product6/2, Product2/2, Product2/1
  Product6/1 -> Sum3/2
  Constant6/1 -> Sum3/1

== system Tricopter_Controlled/TriCopter FCS/Simulink to px4 input/Flat Earth to LLA/ne to lat//long/Latitude Between +//- 90  ==
  mu l : Inport
  Constant1 : Constant  Value=180
  Constant3 : Constant  Value=90
  Constant4 : Constant  Value=180
  Constant5 : Constant  Value=360
  Data Type Conversion : DataTypeConversion
  Demux : Demux  Outputs=2
  Gain : Gain  Gain=180
  Gain1 : Gain  Gain=2
  Gain2 : Gain  Gain=2
  Gain3 : Gain  Gain=360
  Gain4 : Gain  Gain=180
  Logical Operator1 : Logic  AllPortsSameDT=off  OutDataTypeStr=boolean
  Math Function1 : Math  Operator=rem  SaturateOnIntegerOverflow=on
  Math Function2 : Math  Operator=rem  SaturateOnIntegerOverflow=on
  Mux : Mux  Inputs=2
  Product : Product  Inputs=*/  RndMeth=Zero
  Product1 : Product  RndMeth=Zero
  Product2 : Product  Inputs=*/  RndMeth=Zero
  Product3 : Product  RndMeth=Zero
  Rounding Function : Rounding  Operator=fix
  Rounding Function1 : Rounding  Operator=fix
  Rounding Function2 : Rounding  Operator=fix
  Sum1 : Sum  Inputs=|-+
  Sum2 : Sum  Inputs=+--
  Sum3 : Sum  Inputs=++|
  sqrt : Sqrt  AlgorithmType=Newton-Raphson  SaturateOnIntegerOverflow=on
  "mu l " : Outport
  wires:
  Sum3/1 -> Mux/2
  Demux/2 -> Sum3/2
  Demux/1 -> Math Function1/1
  mu l/1 -> Demux/1
  Mux/1 -> "mu l "/1
  Constant1/1 -> Product/2
  Product/1 -> Rounding Function/1, Gain1/1
  Rounding Function/1 -> Gain/1
  Gain/1 -> Sum2/2
  Sum2/1 -> Mux/1
  Constant3/1 -> Math Function2/2
  Math Function2/1 -> Product3/2
  Product3/1 -> Sum2/3
  Rounding Function2/1 -> Gain2/1
  Gain2/1 -> Product3/1, Logical Operator1/1, Logical Operator1/2
  Product1/1 -> sqrt/1
  sqrt/1 -> Rounding Function2/1
  Constant4/1 -> Product2/2
  Product2/1 -> Rounding Function1/1
  Rounding Function1/1 -> Gain3/1
  Gain3/1 -> Sum1/1
  Math Function1/1 -> Sum1/2, Product2/1
  Sum1/1 -> Math Function2/1, Product/1, Sum2/1
  Constant5/1 -> Math Function1/2
  Logical Operator1/1 -> Data Type Conversion/1
  Gain4/1 -> Sum3/1
  Data Type Conversion/1 -> Gain4/1
  Gain1/1 -> Product1/2, Product1/1

== system Tricopter_Controlled/TriCopter FCS/Simulink to px4 input/Flat Earth to LLA/ne to lat//long/LongLat_offset  ==
  XY : Inport
  mu : Inport  Port=2
  " " : Trigonometry
  "  " : Trigonometry  Operator=cos
  Demux : Demux  Outputs=2
  "Find Radian/Distance " : Subsystem  TreatAsAtomicUnit=on
  Mux : Mux  Inputs=2
  Sum : Sum  Inputs=|+-
  Sum1 : Sum  Inputs=|++
  deg2rad : Gain  Gain=pi/180  SaturateOnIntegerOverflow=on  OutDataTypeStr=Inherit: Same as input  ParamDataTypeStr=Inherit: Same as input
  rad lat : Product  RndMeth=Zero
  "rad long " : Product  RndMeth=Zero
  ref_pos : Constant  Value=0
  x*cos : Product  RndMeth=Zero
  x*sin : Product  RndMeth=Zero
  y*cos : Product  RndMeth=Zero
  y*sin : Product  RndMeth=Zero
  DeltaLL_rad : Outport
  wires:
  mu/1 -> "Find Radian/Distance "/1(mu)
  "Find Radian/Distance "/1(dNorth) -> rad lat/2
  "Find Radian/Distance "/2(dEast) -> "rad long "/1
  rad lat/1 -> Mux/1
  "rad long "/1 -> Mux/2
  Mux/1 -> DeltaLL_rad/1
  deg2rad/1 -> "  "/1, " "/1
  Demux/2 -> y*cos/1, y*sin/1
  Sum1/1 -> "rad long "/2
  y*cos/1 -> Sum1/2
  x*sin/1 -> Sum1/1
  Sum/1 -> rad lat/1
  y*sin/1 -> Sum/2
  " "/1 -> x*sin/2, y*sin/2
  x*cos/1 -> Sum/1
  "  "/1 -> y*cos/2, x*cos/2
  Demux/1 -> x*sin/1, x*cos/1
  XY/1 -> Demux/1
  ref_pos/1 -> deg2rad/1

== system Tricopter_Controlled/TriCopter FCS/Simulink to px4 input/Flat Earth to LLA/ne to lat//long/Longitude Between +//-180  ==
  mu l : Inport
  Constant : Constant  Value=180
  Constant2 : Constant  Value=360
  Demux1 : Demux  Outputs=2
  Gain : Gain  Gain=360
  Math Function2 : Math  Operator=rem  SaturateOnIntegerOverflow=on
  Mux1 : Mux  Inputs=2
  Product : Product  Inputs=*/  RndMeth=Zero
  Rounding Function : Rounding  Operator=fix
  Sum2 : Sum  Inputs=|-+
  "mu l " : Outport
  wires:
  Mux1/1 -> "mu l "/1
  Demux1/1 -> Mux1/1
  mu l/1 -> Demux1/1
  Constant/1 -> Product/2
  Product/1 -> Rounding Function/1
  Rounding Function/1 -> Gain/1
  Gain/1 -> Sum2/1
  Sum2/1 -> Mux1/2
  Demux1/2 -> Math Function2/1
  Constant2/1 -> Math Function2/2
  Math Function2/1 -> Product/1, Sum2/2

== system Tricopter_Controlled/TriCopter FCS/TriCopter FCS/Control and guidance/Control allocator/Hover deflections1 ==
  Contro Inputs1 : Constant  Value=Hover_throtle_1
  Contro Inputs2 : Constant  Value=Hover_throtle_23
  Contro Inputs3 : Constant  Value=Hover_eta_23
  Gain : Gain  Gain=-1
  Ground : Ground
  Mux : Mux  Inputs=9
  Trim deflectins : Outport
  wires:
  Contro Inputs1/1 -> Mux/1
  Contro Inputs2/1 -> Mux/7, Mux/4
  Ground/1 -> Mux/2, Mux/6, Mux/9, Mux/3
  Contro Inputs3/1 -> Gain/1, Mux/5
  Gain/1 -> Mux/8
  Mux/1 -> Trim deflectins/1

== system Tricopter_Controlled/TriCopter FCS/TriCopter FCS/Control and guidance/Control allocator/Hover deflections2 ==
  Contro Inputs1 : Constant  Value=Hover_throtle_1
  Contro Inputs2 : Constant  Value=Hover_throtle_23
  Contro Inputs3 : Constant  Value=Hover_eta_23
  Gain : Gain  Gain=-1
  Ground : Ground
  Mux : Mux  Inputs=9
  Trim deflectins : Outport
  wires:
  Contro Inputs1/1 -> Mux/1
  Contro Inputs2/1 -> Mux/7, Mux/4
  Ground/1 -> Mux/2, Mux/6, Mux/9, Mux/3
  Contro Inputs3/1 -> Gain/1, Mux/5
  Gain/1 -> Mux/8
  Mux/1 -> Trim deflectins/1
